simulink model "ref_model"  (R2016b)
settings: Solver=VariableStepAuto  StartTime=0.0  StopTime=StopTime  RelTol=1e-3
values from neighbouring files (symbols this model uses):
  A = 0.1    [constant_cs_varying_ks.m]    (also in constant_ks_varying_cs.m)
  cc = 1649    [constant_cs_varying_ks.m]    (also in constant_ks_varying_cs.m)
  cp = 1360    [constant_cs_varying_ks.m]    (also in constant_ks_varying_cs.m)
  cs = 1650    [constant_cs_varying_ks.m]    (also in constant_ks_varying_cs.m = 500)
  kc = 20000    [constant_cs_varying_ks.m]    (also in constant_ks_varying_cs.m)
  kp = 45005    [constant_cs_varying_ks.m]    (also in constant_ks_varying_cs.m)
  ks = ks + 5000    (= 5000)    [constant_cs_varying_ks.m]    (also in constant_ks_varying_cs.m = 10000)
  kt = 160000    [constant_cs_varying_ks.m]    (also in constant_ks_varying_cs.m)
  m_h = 20    [constant_cs_varying_ks.m]    (also in constant_ks_varying_cs.m)
  m_s = 240    [constant_cs_varying_ks.m]    (also in constant_ks_varying_cs.m)
  m_u = 36    [constant_cs_varying_ks.m]    (also in constant_ks_varying_cs.m)
  omega = 2*pi*f    [constant_cs_varying_ks.m]    (also in constant_ks_varying_cs.m)
settings Model: Creator=Student  LastModifiedBy=Steven

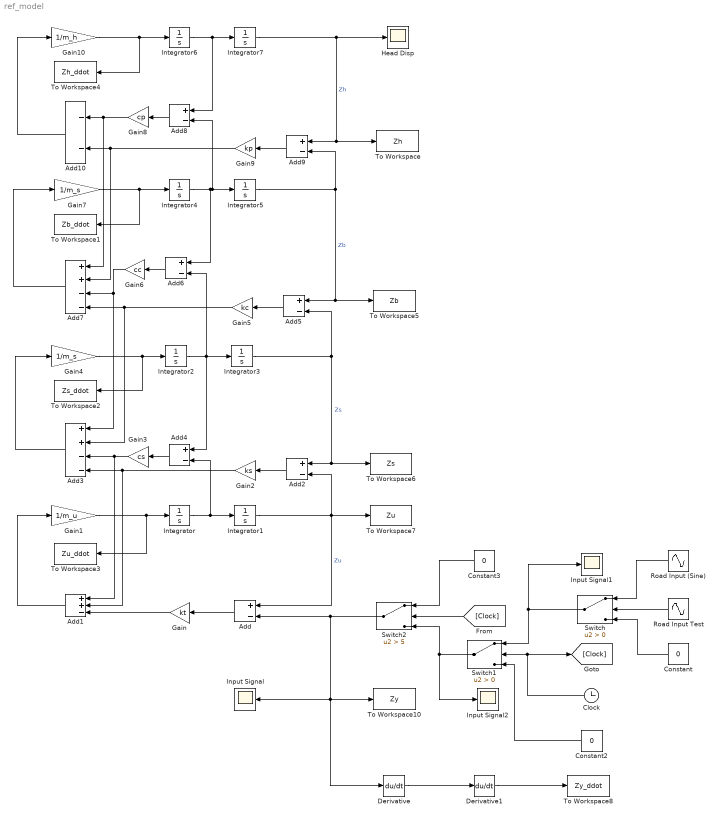
== system ref_model ==
  Add{,2,4..6,8..9} (7 alike) : Sum  Inputs=+-
  Add1 : Sum  Inputs=++-
  Add10 : Sum  Inputs=--
  Add3 : Sum  Inputs=++--
  Add7 : Sum  Inputs=++--
  Clock : Clock
  Constant : Constant  Value=0
  Constant2 : Constant  Value=0
  Constant3 : Constant  Value=0
  Derivative : Derivative
  Derivative1 : Derivative
  Gain : Gain  Gain=kt
  Gain1 : Gain  Gain=1/m_u
  Gain10 : Gain  Gain=1/m_h
  Gain2 : Gain  Gain=ks
  Gain3 : Gain  Gain=cs
  Gain4 : Gain  Gain=1/m_s
  Gain5 : Gain  Gain=kc
  Gain6 : Gain  Gain=cc
  Gain7 : Gain  Gain=1/m_s
  Gain8 : Gain  Gain=cp
  Gain9 : Gain  Gain=kp
  Head Disp : Scope
  Input Signal : Scope
  Input Signal1 : Scope
  Input Signal2 : Scope
  Integrator{,1..7} (8 alike) : Integrator
  Road Input (Sine) : Sin  Amplitude=A  Frequency=omega  SampleTime=0
  Road Input Test : Sin  Amplitude=A  Frequency=omega  SampleTime=0
  Switch : Switch  Criteria=u2 > Threshold
  Switch1 : Switch  Criteria=u2 > Threshold
  Switch2 : Switch  Criteria=u2 > Threshold  Threshold=5
  To Workspace : ToWorkspace  VariableName=Zh  SaveFormat=Timeseries  SampleTime=-1
  To Workspace1 : ToWorkspace  VariableName=Zb_ddot  SaveFormat=Timeseries  SampleTime=-1
  To Workspace10 : ToWorkspace  VariableName=Zy  SaveFormat=Timeseries  SampleTime=-1
  To Workspace2 : ToWorkspace  VariableName=Zs_ddot  SaveFormat=Timeseries  SampleTime=-1
  To Workspace3 : ToWorkspace  VariableName=Zu_ddot  SaveFormat=Timeseries  SampleTime=-1
  To Workspace4 : ToWorkspace  VariableName=Zh_ddot  SaveFormat=Timeseries  SampleTime=-1
  To Workspace5 : ToWorkspace  VariableName=Zb  SaveFormat=Timeseries  SampleTime=-1
  To Workspace6 : ToWorkspace  VariableName=Zs  SaveFormat=Timeseries  SampleTime=-1
  To Workspace7 : ToWorkspace  VariableName=Zu  SaveFormat=Timeseries  SampleTime=-1
  To Workspace8 : ToWorkspace  VariableName=Zy_ddot  SaveFormat=Timeseries  SampleTime=-1
  wires:
  Add/1 -> Gain/1
  Gain/1 -> Add1/3
  Gain3/1 -> Add3/3, Add1/1
  Gain2/1 -> Add3/4, Add1/2
  Add1/1 -> Gain1/1
  Gain1/1 -> To Workspace3/1, Integrator/1
  Integrator/1 -> Add4/2, Integrator1/1
  Integrator1/1 -> Add2/2, To Workspace7/1, Add/1  "Zu"
  Add2/1 -> Gain2/1
  Add4/1 -> Gain3/1
  Gain4/1 -> Integrator2/1, To Workspace2/1
  Integrator2/1 -> Add6/2, Integrator3/1, Add4/1
  Add3/1 -> Gain4/1
  Integrator3/1 -> Add5/2, To Workspace6/1, Add2/1  "Zs"
  Add5/1 -> Gain5/1
  Gain5/1 -> Add7/4, Add3/2
  Add6/1 -> Gain6/1
  Gain6/1 -> Add7/3, Add3/1
  Gain7/1 -> To Workspace1/1, Integrator4/1
  Integrator4/1 -> Add6/1, Add8/2, Integrator5/1
  Add7/1 -> Gain7/1
  Add8/1 -> Gain8/1
  Add9/1 -> Gain9/1
  Integrator5/1 -> Add9/2, Add5/1, To Workspace5/1  "Zb"
  Gain8/1 -> Add10/1, Add7/1
  Gain10/1 -> To Workspace4/1, Integrator6/1
  Integrator6/1 -> Add8/1, Integrator7/1
  Add10/1 -> Gain10/1
  Integrator7/1 -> Head Disp/1, Add9/1, To Workspace/1  "Zh"
  Switch/1 -> Input Signal1/1, Switch1/1
  Gain9/1 -> Add7/2, Add10/2
  Road Input Test/1 -> Switch/2
  Road Input (Sine)/1 -> Switch/1
  Constant/1 -> Switch/3
  Derivative/1 -> Derivative1/1
  Derivative1/1 -> To Workspace8/1
  Constant2/1 -> Switch1/3
  Switch2/1 -> Derivative/1, Input Signal/1, To Workspace10/1, Add/2
  Switch1/1 -> Switch2/3, Input Signal2/1
  Constant3/1 -> Switch2/1
  Clock/1 -> [Clock], Switch1/2
  [Clock] -> Switch2/2
